simulink model "1.3"  (R2018a)
settings: Solver=ode4  StartTime=0.0  StopTime=5  FixedStep=0.001  RelTol=1e-3
undefined symbols (not defined in the file): A, B, L0, L1, L2
settings Model: Creator=80741  LastModifiedBy=80741
settings DataIOCC: LimitDataPoints=on  SaveFormat=Array  SignalLoggingSaveFormat=ModelDataLogs
settings OptimizationCC: InitFltsAndDblsToZero=on  LifeSpan=inf
settings DebuggingCC: SaveWithParameterizedLinksMsg=none  UnderspecifiedInitializationDetection=Classic  MergeDetectMultiDrivingBlocksExec=none  SignalResolutionControl=TryResolveAllWithWarning  SolverPrmCheckMsg=warning  MultiTaskDSMMsg=warning  MultiTaskCondExecSysMsg=none  FcnCallInpInsideContextMsg=warning  SFUnexpectedBacktrackingDiag=warning  SFNoUnconditionalDefaultTransitionDiag=warning  SFExecutionAtInitializationDiag=none
settings HardwareCC: ProdBitPerPointer=32  ProdBitPerSizeT=32  ProdBitPerPtrDiffT=32  ProdLargestAtomicFloat=None  ProdIntDivRoundTo=Undefined  ProdEndianess=Unspecified  ProdWordSize=32  ProdHWDeviceType=32-bit Generic
settings ModelReferenceCC: PropagateSignalLabelsOutOfModel=off
settings CodeAppCC: StateflowObjectComments=on
settings GRTTargetCC: TargetFcnLib=ansi_tfl_tmw.mat  TargetLangStandard=C89/C90 (ANSI)  CombineOutputUpdateFcns=off  GRTInterface=on
settings ConfigComp: CovMetricSettings=dw  CovHtmlReporting=on  CovSaveCumulativeToWorkspaceVar=on  CovSaveSingleToWorkspaceVar=on  CovExternalEMLEnable=off

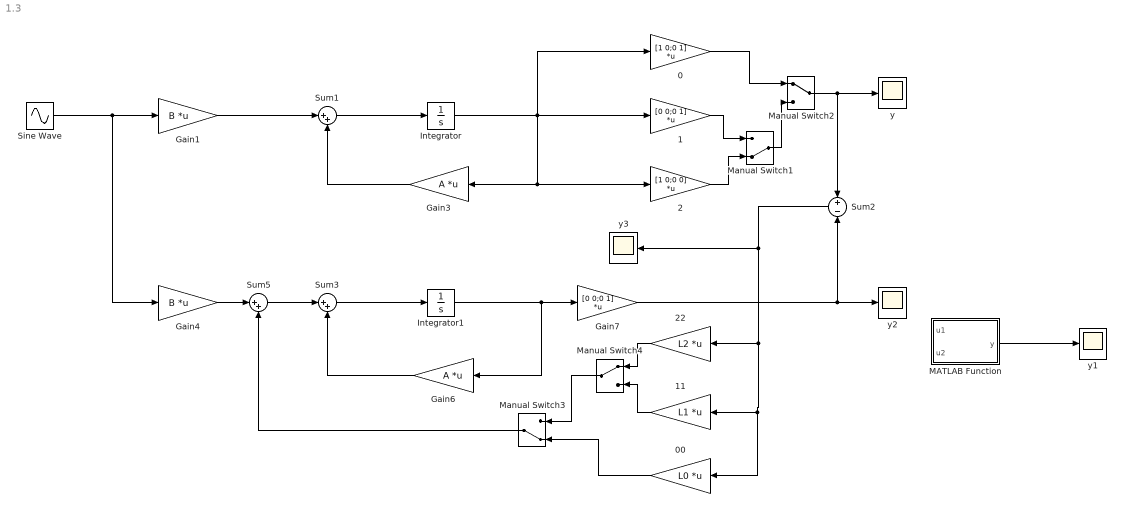
== system 1.3 ==
  0 : Gain  Gain=[1 0;0 1]  Multiplication=Matrix(K*u)
  00 : Gain  Gain=L0  Multiplication=Matrix(K*u)
  "1 " : Gain  Gain=[0 0;0 1]  Multiplication=Matrix(K*u)
  11 : Gain  Gain=L1  Multiplication=Matrix(K*u)
  2 : Gain  Gain=[1 0;0 0]  Multiplication=Matrix(K*u)
  22 : Gain  Gain=L2  Multiplication=Matrix(K*u)
  Gain1 : Gain  Gain=B  Multiplication=Matrix(K*u)
  Gain3 : Gain  Gain=A  Multiplication=Matrix(K*u)
  Gain4 : Gain  Gain=B  Multiplication=Matrix(K*u)
  Gain6 : Gain  Gain=A  Multiplication=Matrix(K*u)
  Gain7 : Gain  Gain=[0 0;0 1]  Multiplication=Matrix(K*u)
  Integrator : Integrator  InitialCondition=[2;1]
  Integrator1 : Integrator
  MATLAB Function : MATLAB Function  TreatAsAtomicUnit=on
  Manual Switch1 : ManualSwitch  CurrentSetting=0
  Manual Switch2 : ManualSwitch
  Manual Switch3 : ManualSwitch  CurrentSetting=0
  Manual Switch4 : ManualSwitch
  Sine Wave : Sin  SampleTime=0
  Sum1 : Sum  Inputs=|++
  Sum2 : Sum  Inputs=+|-
  Sum3 : Sum  Inputs=|++
  Sum5 : Sum  Inputs=|++
  y{,1..3} (4 alike) : Scope
  wires:
  Gain1/1 -> Sum1/1
  Sum1/1 -> Integrator/1
  Integrator/1 -> 0/1, Gain3/1, 2/1, "1 "/1
  Gain4/1 -> Sum5/1
  Sum3/1 -> Integrator1/1
  Integrator1/1 -> Gain7/1, Gain6/1
  Gain6/1 -> Sum3/2
  Sum2/1 -> 00/1, 11/1, 22/1, y3/1
  Sine Wave/1 -> Gain1/1, Gain4/1
  Sum5/1 -> Sum3/1
  Manual Switch3/1 -> Sum5/2
  Gain3/1 -> Sum1/2
  MATLAB Function/1(y) -> y1/1
  "1 "/1 -> Manual Switch1/1
  2/1 -> Manual Switch1/2
  Manual Switch1/1 -> Manual Switch2/2
  0/1 -> Manual Switch2/1
  Manual Switch2/1 -> y/1, Sum2/1
  22/1 -> Manual Switch4/1
  11/1 -> Manual Switch4/2
  Manual Switch4/1 -> Manual Switch3/1
  00/1 -> Manual Switch3/2
  Gain7/1 -> y2/1, Sum2/2

== matlab function 1.3/MATLAB Function ==
  data: u1 input; y output; u2 input
function y = fcn(u1,u2)
y=abs(u1)+abs(u2)
end
